simulink model "model_old"  (R2021b)
settings: Solver=VariableStepAuto  StartTime=0.0  StopTime=10.0  RelTol=1e-3
settings Model: Creator=Vvlad  LastModifiedBy=Vvlad
settings DebuggingCC: UnconnectedInputMsg=none  UnconnectedOutputMsg=none  UnconnectedLineMsg=none
settings RTWCC: DLArmComputeVersion=20.02.1

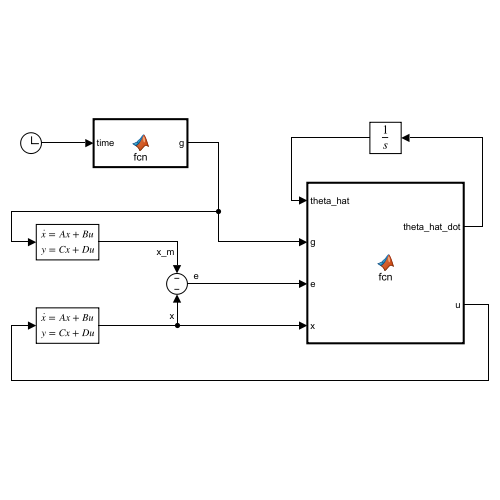
[thumbnail: Simulink's stored preview of the top-level diagram]
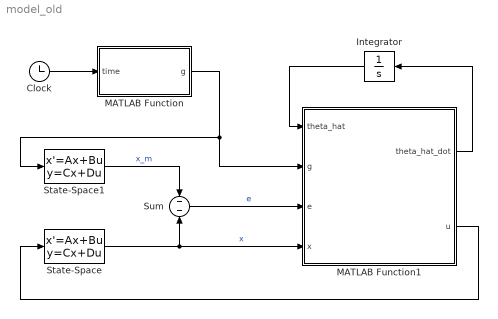
== system model_old ==
  Clock : Clock
  Integrator : Integrator
  MATLAB Function : MATLAB Function  TreatAsAtomicUnit=on
  MATLAB Function1 : MATLAB Function  TreatAsAtomicUnit=on
  State-Space : StateSpace  InitialCondition=0
  State-Space1 : StateSpace  InitialCondition=0
  Sum : Sum  Inputs=--
  wires:
  State-Space1/1 -> Sum/1  "x_m"
  State-Space/1 -> Sum/2, MATLAB Function1/4(x)  "x"
  Clock/1 -> MATLAB Function/1(time)
  MATLAB Function/1(g) -> State-Space1/1, MATLAB Function1/2(g)
  Sum/1 -> MATLAB Function1/3(e)  "e"
  MATLAB Function1/2(u) -> State-Space/1
  MATLAB Function1/1(theta_hat_dot) -> Integrator/1
  Integrator/1 -> MATLAB Function1/1(theta_hat)

== matlab function model_old/MATLAB Function1 ==
  data: theta_hat input; theta_hat_dot output; g input; e input; x input; u output
function [theta_hat_dot, u] = fcn(theta_hat, g, e, x)
theta_hat_dot = 1;
u = 1;

== matlab function model_old/MATLAB Function ==
  data: time input; g output
function g = fcn(time)

g = 2*sign(sin(0.4*time)) + 3;
